simulink model "LabFabSim2022a__10_6_2023"  (R2022a)
settings: Solver=VariableStepAuto  StartTime=0.0  StopTime=400  RelTol=1e-3  EnableMultiTasking=on
model workspace (MAT data in the model file):
  JsonData : timetable (value not decoded)
  M : Simulink.Parameter (value not decoded)
  ROS_trigger = 0
  SL_ROS_VariableLengthArrays_MaxSizes : object (value not decoded)
undefined symbols (not defined in the file): DOS, DOSinitGen, DTP, DTPGen, DTPInitGen, EmptyLocFound, InitCobot, InitCobotReturn, InitializeSLD, InitLEGO, InitVGRproc2, m, MC, MCGen, MCInitGen, MO, MOGen, MOInitGen, n, NetScan, NetScanInitGen, OrderGen, Spying, SpyingInitGen, WS, WSGen, WSInitGen
libraries: sldelib x1
(part 2 of 4)

== system LabFabSim2022a__10_6_2023/NetworkScan ==
  note: Source: SLD --> Destination: Multiple
  note: Entity Gate:
      | set to open when a positive signal value is passed into the control port. Closes when negative.
  note: Recieve signal from Chance-setting Server block for activation signal
  note: Service Time: 50 Timestep
  note: Generates a single entity that causes Network Scan attack (entity generator) to generate one entity
  note: Sets NetScan_id up to 5 and resets to 1 for next NetworkScan attack
  note: On Service Completion: Send a signal to data-logging SimFunctions
  note: Service Time: 40 Timestep
  note: Service Time: 75 Timestep
  note: Service Time: 60 Timestep
  note: Service Time: 55 Timestep
  Display : Display
  Entity Gate : EntityGate  InputPortMessageModes=m,m  OutputPortMessageModes=m
  Entity Generator : EntityGenerator  InputPortMessageModes=m  OutputPortMessageModes=m  GenerationMethod=Event-based  IntergenerationTimeAction=|  GenerateAction=|  AttributeName=NetScan_id  EntityType=Structured  EntityTypeName=NetScanAttack
      IntergenerationTimeAction=|
      | chanceDOS = rand(1,1);
      | if chanceDOS < 0.3
      |     dt = 1
      GenerateAction=|
      | persistent next_id_NetScan
      | 
      | if isempty(next_id_NetScan)
      |     next_id_NetScan = 1;
      |     %set seed for random number generation
      |     rng(12345);
      | end
      | 
      | entity.NetScan_id = next_id_NetScan
      | next_id_NetScan = next_id_NetScan + 1
      | 
      | if entity.NetScan_id == 2
      |     next_id_NetScan = 1
      settings: InputPortMap=u0
  Entity Server : EntityServer  InputPortMessageModes=m  OutputPortMessageModes=m  Capacity=1  ServiceTimeValue=50  ServiceCompleteAction=|
      | sourceID(4); %sld
      | sourceAddress(7); %/sld_node
      | sourceType(1); %motion sensor
      | sourceLocation(1); %Fischertechnik
      | destinationServiceAddress(3); %/status_update (main)
      | destinationServiceType(4); %Order
      | destinationServiceLocation(1); %Fischertechnik
      | accessedNodeAddress(3); 
      | accessedNodeType(2); %Boolean
      | operation(1); %read/write
      | value(44); %none
  Entity Server1 : EntityServer  InputPortMessageModes=m  OutputPortMessageModes=m  Capacity=1  ServiceTimeValue=40  ServiceCompleteAction=|
      | sourceID(4); %sld
      | sourceAddress(7); %/sld_node
      | sourceType(1); %motion sensor
      | sourceLocation(1); %Fischertechnik
      | destinationServiceAddress(2); %/vgr_node
      | destinationServiceType(3); %Reference Switch
      | destinationServiceLocation(1); %Fischertechnik
      | accessedNodeAddress(3); 
      | accessedNodeType(2); %Boolean
      | operation(1); %read/write
      | value(44); %none
  Entity Server2 : EntityServer  InputPortMessageModes=m  OutputPortMessageModes=m  Capacity=1  ServiceTimeValue=75  ServiceCompleteAction=|
      | sourceID(4); %sld
      | sourceAddress(7); %/sld_node
      | sourceType(1); %motion sensor
      | sourceLocation(1); %Fischertechnik
      | destinationServiceAddress(4); %/lego_node
      | destinationServiceType(1); %Motion Sensor
      | destinationServiceLocation(2); %Expansion
      | accessedNodeAddress(4); 
      | accessedNodeType(1); %String
      | operation(1); %read/write
      | value(44); %none
  Entity Server3 : EntityServer  InputPortMessageModes=m  OutputPortMessageModes=m  Capacity=1  ServiceTimeValue=60  ServiceCompleteAction=|
      | sourceID(4); %sld
      | sourceAddress(7); %/sld_node
      | sourceType(1); %motion sensor
      | sourceLocation(1); %Fischertechnik
      | destinationServiceAddress(5); %/listener (cobot)
      | destinationServiceType(5); %next task
      | destinationServiceLocation(2); %Expansion
      | accessedNodeAddress(5); 
      | accessedNodeType(2); %String
      | operation(1); %read/write
      | value(44); %none
  Entity Server4 : EntityServer  InputPortMessageModes=m  OutputPortMessageModes=m  Capacity=1  ServiceTimeValue=55  ServiceCompleteAction=|
      | sourceID(4); %sld
      | sourceAddress(7); %/sld_node
      | sourceType(1); %motion sensor
      | sourceLocation(1); %Fischertechnik
      | destinationServiceAddress(1); %/hbw_node
      | destinationServiceType(4); %order
      | destinationServiceLocation(1); %Fischertechnik
      | accessedNodeAddress(7); 
      | accessedNodeType(2); %String
      | operation(1); %read/write
      | value(44); %none
  Entity Store : EntityStore  InputPortMessageModes=m  OutputPortMessageModes=m  Capacity=3
      settings: OutputPortMap=o4
  Entity Terminator1 : EntityTerminator  InputPortMessageModes=m  NumberEntitiesArrived=on
      settings: OutputPortMap=o0
  InitNetScan : Subsystem
  NetScan : Subsystem  TreatAsAtomicUnit=on
  "Number of Entities Generated from main " : Display
  Simulink Function1 : Subsystem  TreatAsAtomicUnit=on
  Subsystem1 : Subsystem
  wires:
  Simulink Function1/1(Out1) -> Entity Generator/1
  Entity Terminator1/1 -> Display/1
  Entity Generator/1 -> Entity Store/1
  Entity Store/1 -> Entity Gate/2
  Entity Server/1 -> Entity Server1/1
  NetScan/1(Out1) -> Entity Gate/1
  Subsystem1/1(Out1) -> Simulink Function1/1(In1)
  InitNetScan/1(Out1) -> "Number of Entities Generated from main "/1
  Entity Server1/1 -> Entity Server2/1
  Entity Server2/1 -> Entity Server3/1
  Entity Server3/1 -> Entity Server4/1
  Entity Server4/1 -> Entity Terminator1/1
  Entity Gate/1 -> Entity Server/1

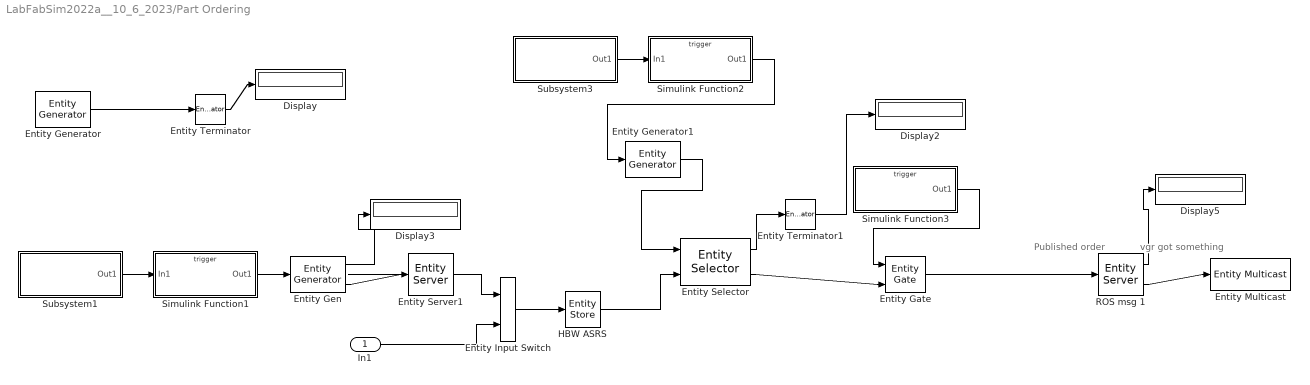
== system LabFabSim2022a__10_6_2023/Part Ordering ==
  note: vgr got something
  note: Published order
  In1 : Inport
  Display{,2..3,5} (4 alike) : Display
  Entity Input Switch : EntityInputSwitch  InputPortMessageModes=m,m  OutputPortMessageModes=m
  Entity Gate : EntityGate  InputPortMessageModes=m,m  OutputPortMessageModes=m  OperatingMode=Release gate  OpenGateAtSimulationStart=on
  "Entity Gen " : EntityGenerator  InputPortMessageModes=m  OutputPortMessageModes=n,m  GenerationMethod=Event-based  GenerateAction=|  AttributeName=PartID|ColorID|ServiceProcess|CurrentStep|CurrentRoute|HBW_ServiceTime|LEGO_ServiceTime|SLD_ServiceTime|HBW_Loc|Rand_seed  AttributeInitialValue=1|1|zeros(1,11)|0|1|zeros(1)|zeros(1)|zeros(1)|zeros(1)|1  NumberEntitiesDeparted=on  EntityType=Structured  EntityTypeName=PartOrder
      | persistent next_id
      | if isempty(next_id)
      |     next_id = 1;
      |     %set seed for random number generation
      |     rng(12345);
      | end
      | 
      | %Assign ID attribute 
      | if next_id <= 9
      |     entity.PartID = next_id;
      |     next_id = next_id + 1
      | end
      | 
      | %Current Step Attribute Setup
      | persistent SEQId;
      | persistent idx2;
      | if isempty(SEQId)
      |     SEQId = 1:15;
      |     idx2 = 1;
      | end
      | if idx2 > numel(SEQId)
      |     idx2 = 1;
      |     entity.PartID = SEQId(idx2);
      | else
      |     entity.PartID = SEQId(idx2);
      | end
      | idx2 = idx2 + 1;
      | entity.CurrentStep=1;
      | 
      | %Randomly Set Order Color 
      | entity.HBW_Loc = randi(3)
      | %To specifically select a part color, uncomment the line below and comment out the line above.
      | %entity.HBW_Loc = 3
      | switch(entity.HBW_Loc)
      |     case 1 
      |         entity.ColorID = 1;
      |         %entity.Color = "red";
      |         %red part ordered
      |     case 2
      |         entity.ColorID = 2;
      |         %entity.Color = "blue";
      |         %blue part ordered 
      |     case 3 
      |         entity.ColorID = 3;
      |         %entity.Color = "white";
      |         %white part ordered 
      | end
      | 
      | %Entity attribute based on color ID
      | if entity.ColorID == 1
      |     entity.ServiceProcess = [2 3 4 5 6 7 8 9 10 11 1];
      |     entity.HBW_ServiceTime = [5];
      |     entity.LEGO_ServiceTime = [4];
      |     entity.SLD_ServiceTime = [5];
      |     
      | else if entity.ColorID == 2
      |     entity.ServiceProcess = [2 3 4 5 6 7 8 9 10 11 1];
      |     entity.HBW_ServiceTime = [6];
      |     entity.LEGO_ServiceTime = [4];
      |     entity.SLD_ServiceTime = [4];
      |     
      | else if entity.ColorID == 3
      |     entity.ServiceProcess = [2 3 4 5 6 7 8 9 10 11 1];
      |     entity.HBW_ServiceTime = [5];
      |     entity.LEGO_ServiceTime = [6];
      |     entity.SLD_ServiceTime = [6];
      | end
      | end
      | 
      | entity.Rand_seed = 123457;
      settings: InputPortMap=u0  OutputPortMap=o0,o3
  Entity Generator : EntityGenerator  OutputPortMessageModes=m  Period=inf  AttributeName=data  EntityType=Structured  EntityTypeName=InitOrders
  Entity Generator1 : EntityGenerator  InputPortMessageModes=m  OutputPortMessageModes=m  GenerationMethod=Event-based  GenerateAction=entity.PartID = randi(9);  AttributeName=PartID  AttributeInitialValue=zeros(1)  EntityType=Structured  EntityTypeName=Order
      settings: InputPortMap=u0
  Entity Multicast : EntityMulticast  Tag=Order  InputPortMessageModes=m  MulticastTag=Order
  Entity Selector : sldelib/Entity Selector  mNumberOfStreams=1  mKeyEntityAttributeName={'PartID'}  mEntityAttributeName={'PartID'}  mMatchingNumberSource=Dialog  mNumberOfMatches=1  mNumberOfMatchesAttribute=Name  mNumEntitiesDepOpt=off  mNumEntitiesInBlockOpt=off  mNumEntitiesExtractedOpt=off
      settings: SourceProductBaseCode=SE
  Entity Server1 : EntityServer  InputPortMessageModes=m  OutputPortMessageModes=m  Capacity=1  ServiceTimeValue=0
  Entity Terminator : EntityTerminator  InputPortMessageModes=m  EntryAction=|  NumberEntitiesArrived=on
      | EntityGen();
      | EntityGen();
      | EntityGen();
      | EntityGen();
      | EntityGen();
      | EntityGen();
      | EntityGen();
      | EntityGen();
      | EntityGen();
      | 
      | %Initially set attack Routers to closed state
      | DOS_Router(2);
      | NetScan_Router(2);
      | Spying_Router(2);
      | DTP_Router(2);
      | MO_Router(2);
      | WS_Router(2);
      | MC_Router(2);
      settings: OutputPortMap=o0
  Entity Terminator1 : EntityTerminator  InputPortMessageModes=m  NumberEntitiesArrived=on
      settings: OutputPortMap=o0
  HBW ASRS : EntityStore  InputPortMessageModes=m  OutputPortMessageModes=m  Capacity=9  EntryAction=OrderGen();
      settings: OutputPortMap=o4
  ROS msg 1 : EntityServer  InputPortMessageModes=m  OutputPortMessageModes=n,m  Capacity=1  ServiceTimeSource=MATLAB action  ServiceTimeValue=0.07  ServiceTimeAction=|  EntryAction=|  ExitAction=|  NumberEntitiesDeparted=on
      ServiceTimeAction=|
      | dt=0
      | persistent rngInit;
      | if isempty(rngInit)
      |     seed = entity.Rand_seed;
      |     rng(seed);
      |     rngInit = true;
      | end
      | 
      | if entity.ColorID == 1 %red
      |     % Pattern: Uniform distribution
      |     % m: Minimum, M: Maximum
      |     m = 0.0253; M = 0.09114;
      |     dt = m + (M - m) * rand;
      | elseif entity.ColorID == 2 %blue
      |     m = 0.05309; M = 0.1517;
      |     dt = m + (M - m) * rand;
      | elseif entity.ColorID == 3 %white
      |     m = 0.06431; M = 0.24846;
      |     dt = m + (M - m) * rand;
      | end
      EntryAction=|
      | sourceID(3); %main
      | sourceAddress(6); %/order
      | sourceType(4); %order
      | sourceLocation(3); %SCADA system
      | destinationServiceAddress(1); %/hbw_node
      | destinationServiceType(4); %order
      | destinationServiceLocation(1); %Fischertechnik
      | accessedNodeAddress(7); 
      | accessedNodeType(1); %String
      | operation(3); %notify-callback
      | value(41); %Published order
      ExitAction=|
      | sourceID(3); %main
      | sourceAddress(2); %/vgr_node
      | sourceType(4); %order
      | sourceLocation(3); %SCADA system
      | destinationServiceAddress(2); %/vgr_node
      | destinationServiceType(4); %order
      | destinationServiceLocation(1); %Fischertechnik
      | accessedNodeAddress(3); 
      | accessedNodeType(1); %String
      | operation(3); %notify-callback
      | value(28); %Published order
      settings: OutputPortMap=o0,o9
  Simulink Function1 : Subsystem  TreatAsAtomicUnit=on
  Simulink Function2 : Subsystem  TreatAsAtomicUnit=on
  Simulink Function3 : Subsystem  TreatAsAtomicUnit=on
  Subsystem1 : Subsystem
  Subsystem3 : Subsystem
  wires:
  Entity Terminator/1 -> Display/1
  Subsystem1/1(Out1) -> Simulink Function1/1(In1)
  Simulink Function1/1(Out1) -> "Entity Gen "/1
  HBW ASRS/1 -> Entity Selector/2
  Simulink Function3/1(Out1) -> Entity Gate/1
  ROS msg 1/2 -> Entity Multicast/1
  ROS msg 1/1 -> Display5/1
  "Entity Gen "/1 -> Display3/1
  "Entity Gen "/2 -> Entity Server1/1
  In1/1 -> Entity Input Switch/2
  Entity Selector/1 -> Entity Terminator1/1
  Entity Generator1/1 -> Entity Selector/1
  Subsystem3/1(Out1) -> Simulink Function2/1(In1)
  Simulink Function2/1(Out1) -> Entity Generator1/1
  Entity Terminator1/1 -> Display2/1
  Entity Generator/1 -> Entity Terminator/1
  Entity Input Switch/1 -> HBW ASRS/1
  Entity Server1/1 -> Entity Input Switch/1
  Entity Selector/2 -> Entity Gate/2
  Entity Gate/1 -> ROS msg 1/1

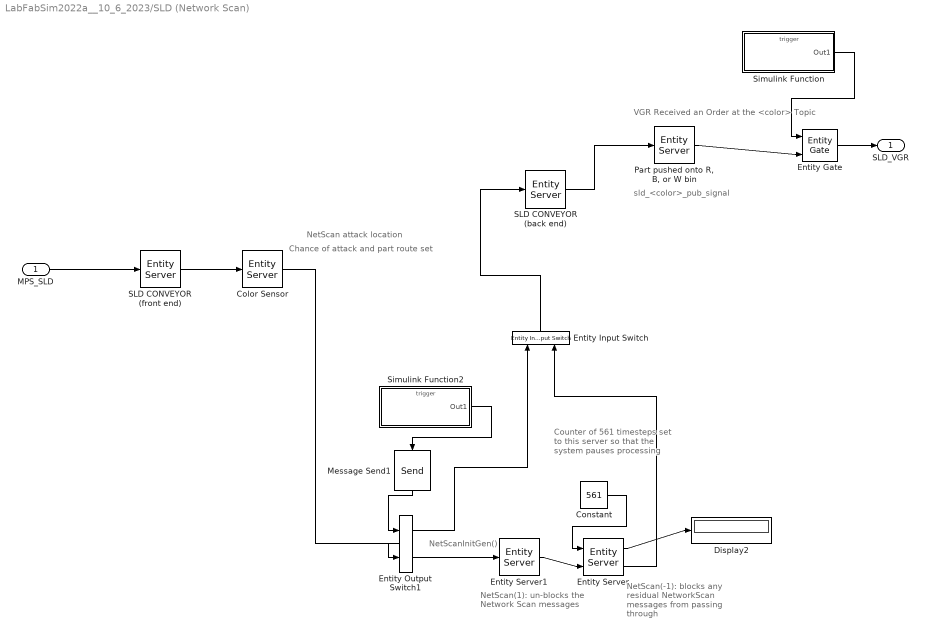
== system LabFabSim2022a__10_6_2023/SLD (Network Scan) ==
  note: VGR Received an Order at the <color> Topic
  note: sld_<color>_pub_signal
  note: NetScanInitGen()
  note: NetScan(1):
      | un-blocks the Network Scan messages
  note: NetScan(-1):
      | blocks any residual NetworkScan messages from passing through
  note: Counter of 561 timesteps set to this server so that the system pauses processing
  note: Chance of attack and part route set
  note: NetScan attack location
  MPS_SLD : Inport
  Color Sensor : EntityServer  InputPortMessageModes=m  OutputPortMessageModes=m  Capacity=1  ServiceTimeValue=0  ExitAction=|
      | chanceNetScan = rand(1,1)
      | if chanceNetScan < 0.0
      |     %Attack Happening!
      |     NetScan_Router(1);
      | 
      | else
      |     %Normal Behavior
      |     NetScan(-1);
      |     NetScan_Router(2);
      | end
  Constant : Constant  Value=561
  Display2 : Display
  Entity Input Switch : EntityInputSwitch  InputPortMessageModes=m,m  OutputPortMessageModes=m
  Entity Output Switch1 : EntityOutputSwitch  InputPortMessageModes=m,m  OutputPortMessageModes=m,m  SwitchingCriterion=From control port  SwitchAttributeName=Attribute1
      settings: InputPortMap=u0,u1
  Entity Gate : EntityGate  InputPortMessageModes=m,m  OutputPortMessageModes=m  OperatingMode=Release gate
  Entity Server : EntityServer  InputPortMessageModes=n,m  OutputPortMessageModes=n,m  Capacity=1  ServiceTimeSource=Signal port  ExitAction=NetScan(-1);  NumberEntitiesDeparted=on
      settings: InputPortMap=u0,u2  OutputPortMap=o0,o9
  Entity Server1 : EntityServer  InputPortMessageModes=m  OutputPortMessageModes=m  Capacity=1  EntryAction=NetScanInitGen();  ServiceCompleteAction=NetScan(1);
  Message Send1 : Send  OutputPortMessageModes=m
  "Part pushed onto R, B, or W bin" : EntityServer  InputPortMessageModes=m  OutputPortMessageModes=m  Capacity=1  ServiceTimeSource=MATLAB action  ServiceTimeAttributeName=SLD_ServiceTime  ServiceTimeAction=|  EntryAction=InitVGRproc2();  ExitAction=|
      ServiceTimeAction=|
      | dt=0
      | persistent rngInit;
      | if isempty(rngInit)
      |     seed = entity.Rand_seed;
      |     rng(seed);
      |     rngInit = true;
      | end
      | 
      | if entity.ColorID == 1 %red
      |     % Pattern: Uniform distribution
      |     % m: Minimum, M: Maximum
      |     m = 5.806; M = 12.40431;
      |     dt = m + (M - m) * rand;
      | elseif entity.ColorID == 2 %blue
      |     m = 13.70771; M = 15.54878;
      |     dt = m + (M - m) * rand;
      | elseif entity.ColorID == 3 %white
      |     m = 1.09164; M = 5.1134;
      |     dt = m + (M - m) * rand;
      | end
      ExitAction=|
      | sourceID(4); %sld
      | sourceAddress(7); %/vgr_node
      | sourceType(1); %motion sensor
      | sourceLocation(1); %Fischertechnik
      | destinationServiceAddress(2); %/vgr_node
      | destinationServiceType(5); %next task
      | destinationServiceLocation(1); %Fischertechnik
      | accessedNodeAddress(3); 
      | accessedNodeType(2); %String
      | operation(3); %notify-callback
      | 
      | if entity.ColorID == 1
      |     value(19); %VGR Received an Order at the RED Topic
      | else if entity.ColorID == 2
      |     value(18); %VGR Received an Order at the BLUE Topic
      | else    
      |     value(20); %VGR Received an Order at the WHITE Topic
      | end
  SLD CONVEYOR (back end) : EntityServer  InputPortMessageModes=m  OutputPortMessageModes=m  Capacity=1  ServiceTimeSource=Attribute  ServiceTimeAttributeName=SLD_ServiceTime
  SLD CONVEYOR (front end) : EntityServer  InputPortMessageModes=m  OutputPortMessageModes=m  Capacity=1  ServiceTimeValue=5
  Simulink Function : Subsystem  TreatAsAtomicUnit=on
  Simulink Function2 : Subsystem  TreatAsAtomicUnit=on
  SLD_VGR : Outport
  wires:
  MPS_SLD/1 -> SLD CONVEYOR (front end)/1
  SLD CONVEYOR (front end)/1 -> Color Sensor/1
  SLD CONVEYOR (back end)/1 -> "Part pushed onto R, B, or W bin"/1
  "Part pushed onto R, B, or W bin"/1 -> Entity Gate/2
  Entity Gate/1 -> SLD_VGR/1
  Simulink Function/1(Out1) -> Entity Gate/1
  Entity Server/1 -> Display2/1
  Entity Server1/1 -> Entity Server/2
  Entity Server/2 -> Entity Input Switch/2
  Color Sensor/1 -> Entity Output Switch1/2
  Entity Input Switch/1 -> SLD CONVEYOR (back end)/1
  Constant/1 -> Entity Server/1
  Message Send1/1 -> Entity Output Switch1/1
  Entity Output Switch1/2 -> Entity Server1/1
  Entity Output Switch1/1 -> Entity Input Switch/1
  Simulink Function2/1(Out1) -> Message Send1/1

== system LabFabSim2022a__10_6_2023/Spying ==
  note: Source: hbw --> Destination: (2,5)
  note: Entity Gate:
      | set to open when a positive signal value is passed into the control port. Closes when negative.
  note: Recieve signal from Chance-setting Server block for activation signal
  note: Service Time: 50 Timestep
  note: Generates a single entity that causes Spying attack (entity generator) to generate one entity
  note: Sets Spying_id up to 5 and resets to 1 for next Spying attack
  note: On Service Completion: Send a signal to data-logging SimFunctions
  note: Service Time: 110 Timestep
  note: Service Time: 75 Timestep
  note: Service Time: 95 Timestep
  note: Service Time: 150 Timestep
  Display : Display
  Entity Gate : EntityGate  InputPortMessageModes=m,m  OutputPortMessageModes=m
  Entity Generator : EntityGenerator  InputPortMessageModes=m  OutputPortMessageModes=m  GenerationMethod=Event-based  IntergenerationTimeAction=|  GenerateAction=|  AttributeName=Spying_id  EntityType=Structured  EntityTypeName=SpyingAttack
      IntergenerationTimeAction=|
      | chanceDOS = rand(1,1);
      | if chanceDOS < 0.3
      |     dt = 1
      GenerateAction=|
      | persistent next_id_Spying
      | 
      | if isempty(next_id_Spying)
      |     next_id_Spying = 1;
      |     %set seed for random number generation
      |     rng(12345);
      | end
      | 
      | entity.Spying_id = next_id_Spying
      | next_id_Spying = next_id_Spying + 1
      | 
      | if entity.Spying_id == 5
      |     next_id_Spying = 1
      settings: InputPortMap=u0
  Entity Server : EntityServer  InputPortMessageModes=m  OutputPortMessageModes=m  Capacity=1  ServiceTimeValue=50  ServiceCompleteAction=|
      | sourceID(1); %hbw
      | sourceAddress(1); %/hbw_node
      | sourceType(5); %next_task
      | sourceLocation(1); %Fischertechnik
      | destinationServiceAddress(2); %/vgr_node
      | destinationServiceType(1); %Motion Sensor
      | destinationServiceLocation(1); %Fischertechnik
      | accessedNodeAddress(3); 
      | accessedNodeType(2); %Boolean
      | operation(1); %read/write
      | value(45); %Spy
  Entity Server1 : EntityServer  InputPortMessageModes=m  OutputPortMessageModes=m  Capacity=1  ServiceTimeValue=110  ServiceCompleteAction=|
      | sourceID(1); %hbw
      | sourceAddress(1); %/hbw_node
      | sourceType(5); %next_task
      | sourceLocation(1); %Fischertechnik
      | destinationServiceAddress(5); %/lego_node
      | destinationServiceType(1); %Motion Sensor
      | destinationServiceLocation(2); %Expansion
      | accessedNodeAddress(5); 
      | accessedNodeType(2); %Boolean
      | operation(1); %read/write
      | value(45); %Spy
  Entity Server2 : EntityServer  InputPortMessageModes=m  OutputPortMessageModes=m  Capacity=1  ServiceTimeValue=75  ServiceCompleteAction=|
      | sourceID(1); %hbw
      | sourceAddress(1); %/hbw_node
      | sourceType(5); %next_task
      | sourceLocation(1); %Fischertechnik
      | destinationServiceAddress(2); %/vgr_node
      | destinationServiceType(1); %Motion Sensor
      | destinationServiceLocation(1); %Fischertechnik
      | accessedNodeAddress(3); 
      | accessedNodeType(2); %Boolean
      | operation(1); %read/write
      | value(45); %Spy
  Entity Server3 : EntityServer  InputPortMessageModes=m  OutputPortMessageModes=m  Capacity=1  ServiceTimeValue=95  ServiceCompleteAction=|
      | sourceID(1); %hbw
      | sourceAddress(1); %/hbw_node
      | sourceType(5); %next_task
      | sourceLocation(1); %Fischertechnik
      | destinationServiceAddress(5); %/lego_node
      | destinationServiceType(1); %Motion Sensor
      | destinationServiceLocation(2); %Expansion
      | accessedNodeAddress(5);  
      | accessedNodeType(2); %Boolean
      | operation(1); %read/write
      | value(45); %Spy
  Entity Server4 : EntityServer  InputPortMessageModes=m  OutputPortMessageModes=m  Capacity=1  ServiceTimeValue=150  ServiceCompleteAction=|
      | sourceID(1); %hbw
      | sourceAddress(1); %/hbw_node
      | sourceType(5); %next_task
      | sourceLocation(1); %Fischertechnik
      | destinationServiceAddress(5); %/lego_node
      | destinationServiceType(1); %Motion Sensor
      | destinationServiceLocation(2); %Expansion
      | accessedNodeAddress(5);  
      | accessedNodeType(2); %Boolean
      | operation(1); %read/write
      | value(45); %Spy
  Entity Store : EntityStore  InputPortMessageModes=m  OutputPortMessageModes=m  Capacity=6
      settings: OutputPortMap=o4
  Entity Terminator1 : EntityTerminator  InputPortMessageModes=m  NumberEntitiesArrived=on
      settings: OutputPortMap=o0
  InitSpying : Subsystem
  "Number of Entities Generated from main " : Display
  Simulink Function1 : Subsystem  TreatAsAtomicUnit=on
  Spying : Subsystem  TreatAsAtomicUnit=on
  Subsystem1 : Subsystem
  wires:
  Simulink Function1/1(Out1) -> Entity Generator/1
  Entity Terminator1/1 -> Display/1
  Entity Generator/1 -> Entity Store/1
  Entity Store/1 -> Entity Gate/2
  Entity Server/1 -> Entity Server1/1
  Spying/1(Out1) -> Entity Gate/1
  Subsystem1/1(Out1) -> Simulink Function1/1(In1)
  InitSpying/1(Out1) -> "Number of Entities Generated from main "/1
  Entity Server1/1 -> Entity Server2/1
  Entity Server2/1 -> Entity Server3/1
  Entity Server3/1 -> Entity Server4/1
  Entity Server4/1 -> Entity Terminator1/1
  Entity Gate/1 -> Entity Server/1

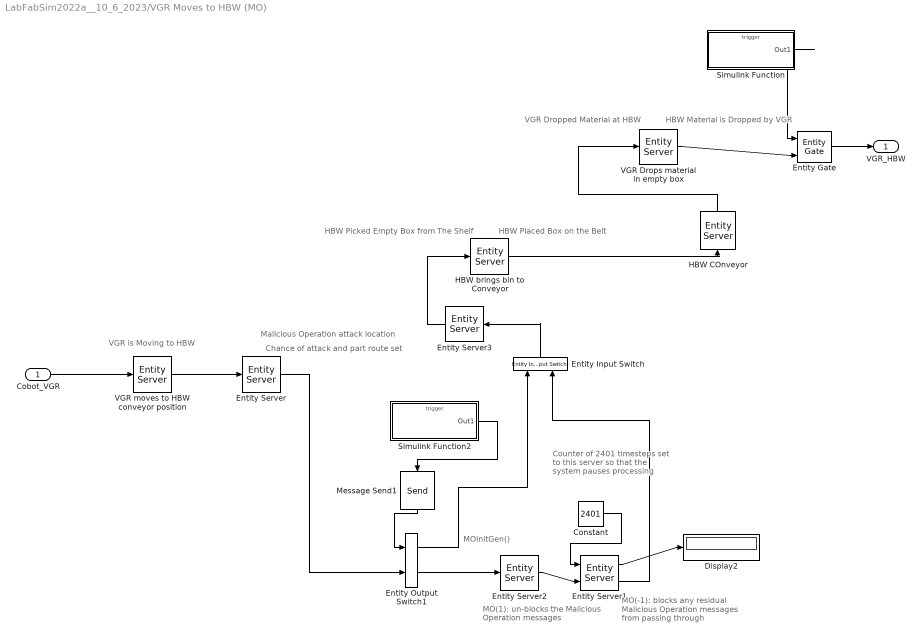
== system LabFabSim2022a__10_6_2023/VGR Moves to HBW (MO) ==
  note: HBW Material is Dropped by VGR
  note: VGR Dropped Material at HBW
  note: HBW Placed Box on the Belt
  note: HBW Picked Empty Box from The Shelf
  note: VGR is Moving to HBW
  note: MOInitGen()
  note: MO(-1):
      | blocks any residual Malicious Operation messages from passing through
  note: MO(1):
      | un-blocks the Malicious Operation messages
  note: Counter of 2401 timesteps set to this server so that the system pauses processing
  note: Malicious Operation attack location
  note: Chance of attack and part route set
  Cobot_VGR : Inport
  Constant : Constant  Value=2401
  Display2 : Display
  Entity Input Switch : EntityInputSwitch  InputPortMessageModes=m,m  OutputPortMessageModes=m
  Entity Output Switch1 : EntityOutputSwitch  InputPortMessageModes=m,m  OutputPortMessageModes=m,m  SwitchingCriterion=From control port  SwitchAttributeName=Attribute1
      settings: InputPortMap=u0,u1
  Entity Gate : EntityGate  InputPortMessageModes=m,m  OutputPortMessageModes=m  OperatingMode=Release gate
  Entity Server : EntityServer  InputPortMessageModes=m  OutputPortMessageModes=m  Capacity=1  ServiceTimeValue=0  ExitAction=|
      | chanceMO = rand(1,1)
      | if chanceMO < 0.0
      |     %Attack Happening!
      |     MO_Router(1);
      | 
      | else
      |     %Normal Behavior
      |     MO(-1);
      |     MO_Router(2);
      | end
  Entity Server1 : EntityServer  InputPortMessageModes=n,m  OutputPortMessageModes=n,m  Capacity=1  ServiceTimeSource=Signal port  ExitAction=MO(-1);  NumberEntitiesDeparted=on
      settings: InputPortMap=u0,u2  OutputPortMap=o0,o9
  Entity Server2 : EntityServer  InputPortMessageModes=m  OutputPortMessageModes=m  Capacity=1  EntryAction=MOInitGen();  ServiceCompleteAction=MO(1);
  Entity Server3 : EntityServer  InputPortMessageModes=m  OutputPortMessageModes=m  Capacity=1  ServiceTimeSource=MATLAB action  ServiceTimeAction=|
      | dt=0
      | persistent rngInit;
      | if isempty(rngInit)
      |     seed = entity.Rand_seed;
      |     rng(seed);
      |     rngInit = true;
      | end
      | 
      | if entity.ColorID == 1 %red
      |     % Pattern: Uniform distribution
      |     % m: Minimum, M: Maximum
      |     m = 9.7679; M = 9.7679;
      |     dt = m + (M - m) * rand;
      | elseif entity.ColorID == 2 %blue
      |     m = 6.5315; M = 7.32;
      |     dt = m + (M - m) * rand;
      | elseif entity.ColorID == 3 %white
      |     m = 13.1578; M = 13.8905;
      |     dt = m + (M - m) * rand;
      | end
  HBW COnveyor : EntityServer  InputPortMessageModes=m  OutputPortMessageModes=m  Capacity=1  ServiceTimeSource=MATLAB action  ServiceTimeAction=|
      | dt=0
      | persistent rngInit;
      | if isempty(rngInit)
      |     seed = entity.Rand_seed;
      |     rng(seed);
      |     rngInit = true;
      | end
      | 
      | if entity.ColorID == 1 %red
      |     % Pattern: Uniform distribution
      |     % m: Minimum, M: Maximum
      |     m = 0.0599; M = 0.7454;
      |     dt = m + (M - m) * rand;
      | elseif entity.ColorID == 2 %blue
      |     m = 0.6055; M = 0.6167;
      |     dt = m + (M - m) * rand;
      | elseif entity.ColorID == 3 %white
      |     m = 0.6407; M = 0.6611;
      |     dt = m + (M - m) * rand;
      | end
  HBW brings bin to Conveyor : EntityServer  InputPortMessageModes=m  OutputPortMessageModes=m  Capacity=1  ServiceTimeSource=MATLAB action  ServiceTimeValue=3  ServiceTimeAttributeName=HBW_ServiceTime  ServiceTimeAction=|  EntryAction=|  ExitAction=|
      ServiceTimeAction=|
      | dt=0
      | persistent rngInit;
      | if isempty(rngInit)
      |     seed = entity.Rand_seed;
      |     rng(seed);
      |     rngInit = true;
      | end
      | 
      | if entity.ColorID == 1 %red
      |     % Pattern: Uniform distribution
      |     % m: Minimum, M: Maximum
      |     m = 20.0831; M = 20.9407;
      |     dt = m + (M - m) * rand;
      | elseif entity.ColorID == 2 %blue
      |     m = 17.0487; M = 17.2651;
      |     dt = m + (M - m) * rand;
      | elseif entity.ColorID == 3 %white
      |     m = 23.2158; M = 24.0842;
      |     dt = m + (M - m) * rand;
      | end
      EntryAction=|
      | sourceID(1); %hbw
      | sourceAddress(1); %/hbw_node
      | sourceType(3); %reference switch
      | sourceLocation(1); %Fischertechnik
      | destinationServiceAddress(1); %/hbw_node
      | destinationServiceType(5); %next task
      | destinationServiceLocation(1); %Fischertechnik
      | accessedNodeAddress(1); 
      | accessedNodeType(1); %String
      | operation(3); %notify-callback
      | value(4); %HBW Picked Empty Box from The Shelf
      ExitAction=|
      | sourceID(1); %hbw
      | sourceAddress(1); %/hbw_node
      | sourceType(1); %Motion Sensor
      | sourceLocation(1); %Fischertechnik
      | destinationServiceAddress(1); %/hbw_node
      | destinationServiceType(5); %next task
      | destinationServiceLocation(1); %Fischertechnik
      | accessedNodeAddress(1); 
      | accessedNodeType(1); %String
      | operation(3); %notify-callback
      | value(6); %HBW Placed Box on the Belt
  Message Send1 : Send  OutputPortMessageModes=m
  Simulink Function : Subsystem  TreatAsAtomicUnit=on
  Simulink Function2 : Subsystem  TreatAsAtomicUnit=on
  VGR Drops material in empty box : EntityServer  InputPortMessageModes=m  OutputPortMessageModes=m  Capacity=1  ServiceTimeSource=MATLAB action  ServiceTimeValue=6  ServiceTimeAttributeName=HBW_ServiceTime  ServiceTimeAction=|  EntryAction=|  ExitAction=|
      ServiceTimeAction=|
      | dt=0
      | persistent rngInit;
      | if isempty(rngInit)
      |     seed = entity.Rand_seed;
      |     rng(seed);
      |     rngInit = true;
      | end
      | 
      | if entity.ColorID == 1 %red
      |     % Pattern: Uniform distribution
      |     % m: Minimum, M: Maximum
      |     m = 6.1187; M = 6.3253;
      |     dt = m + (M - m) * rand;
      | elseif entity.ColorID == 2 %blue
      |     m = 6.3414; M = 6.4349;
      |     dt = m + (M - m) * rand;
      | elseif entity.ColorID == 3 %white
      |     m = 6.3623; M = 6.4411;
      |     dt = m + (M - m) * rand;
      | end
      EntryAction=|
      | BinSupplied();
      | 
      | sourceID(1); %hbw
      | sourceAddress(1); %/hbw_node
      | sourceType(1); %Motion Sensor 
      | sourceLocation(1); %Fischertechnik
      | destinationServiceAddress(2); %/vgr_node
      | destinationServiceType(5); %next task
      | destinationServiceLocation(1); %Fischertechnik
      | accessedNodeAddress(3); 
      | accessedNodeType(2); %Boolean
      | operation(3); %notify-callback
      | value(21); %VGR Dropped Material at HBW
      ExitAction=|
      | sourceID(1); %hbw
      | sourceAddress(1); %/hbw_node
      | sourceType(5); %next task
      | sourceLocation(1); %Fischertechnik
      | destinationServiceAddress(1); %/hbw_node
      | destinationServiceType(5); %next task
      | destinationServiceLocation(1); %Fischertechnik
      | accessedNodeAddress(1); 
      | accessedNodeType(1); %String
      | operation(3); %notify-callback
      | value(8); %HBW Material is Dropped by VGR
  VGR moves to HBW conveyor position : EntityServer  InputPortMessageModes=m  OutputPortMessageModes=m  Capacity=1  ServiceTimeSource=MATLAB action  ServiceTimeValue=3  ServiceTimeAction=|  ServiceCompleteAction=|
      ServiceTimeAction=|
      | dt=0
      | persistent rngInit;
      | if isempty(rngInit)
      |     seed = entity.Rand_seed;
      |     rng(seed);
      |     rngInit = true;
      | end
      | 
      | if entity.ColorID == 1 %red
      |     % Pattern: Uniform distribution
      |     % m: Minimum, M: Maximum
      |     m = 9.1993; M = 9.5444;
      |     dt = m + (M - m) * rand;
      | elseif entity.ColorID == 2 %blue
      |     m = 8.5836; M = 9.294;
      |     dt = m + (M - m) * rand;
      | elseif entity.ColorID == 3 %white
      |     m = 9.1114; M = 9.2737;
      |     dt = m + (M - m) * rand;
      | end
      ServiceCompleteAction=|
      | sourceID(3); %main
      | sourceAddress(6); %/order
      | sourceType(5); %next task
      | sourceLocation(1); %Fischer
      | destinationServiceAddress(2); %/vgr_node
      | destinationServiceType(5); %next task
      | destinationServiceLocation(1); %Fischertechnik
      | accessedNodeAddress(3); 
      | accessedNodeType(1); %String
      | operation(3); %notify-callback
      | value(29); %vgr is moving to hbw
  VGR_HBW : Outport
  wires:
  VGR moves to HBW conveyor position/1 -> Entity Server/1
  Cobot_VGR/1 -> VGR moves to HBW conveyor position/1
  Entity Gate/1 -> VGR_HBW/1
  Simulink Function/1(Out1) -> Entity Gate/1
  VGR Drops material in empty box/1 -> Entity Gate/2
  HBW brings bin to Conveyor/1 -> HBW COnveyor/1
  Entity Server1/1 -> Display2/1
  Constant/1 -> Entity Server1/1
  Entity Input Switch/1 -> Entity Server3/1
  Entity Server/1 -> Entity Output Switch1/2
  Entity Output Switch1/2 -> Entity Server2/1
  Simulink Function2/1(Out1) -> Message Send1/1
  Entity Server2/1 -> Entity Server1/2
  Entity Server1/2 -> Entity Input Switch/2
  Message Send1/1 -> Entity Output Switch1/1
  Entity Output Switch1/1 -> Entity Input Switch/1
  Entity Server3/1 -> HBW brings bin to Conveyor/1
  HBW COnveyor/1 -> VGR Drops material in empty box/1

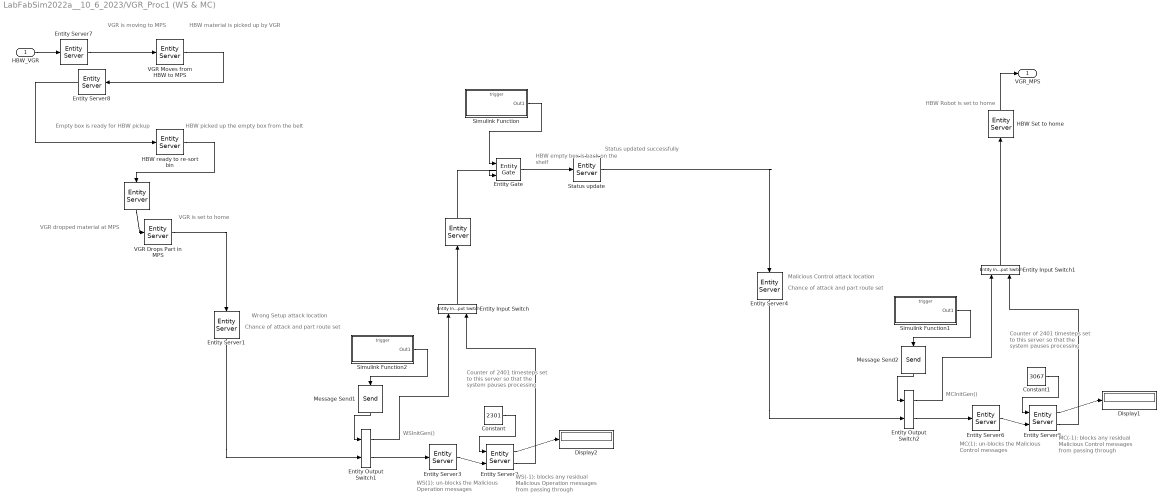
== system LabFabSim2022a__10_6_2023/VGR_Proc1 (WS & MC) ==
  note: Status updated successfully
  note: HBW empty box is back on the shelf
  note: HBW Robot is set to home
  note: VGR is set to home
  note: VGR dropped material at MPS
  note: HBW picked up the empty box from the belt
  note: Empty box is ready for HBW pickup
  note: HBW material is picked up by VGR
  note: VGR is moving to MPS
  note: WS(-1):
      | blocks any residual Malicious Operation messages from passing through
  note: Counter of 2401 timesteps set to this server so that the system pauses processing
  note: Chance of attack and part route set
  note: WSInitGen()
  note: WS(1):
      | un-blocks the Malicious Operation messages
  note: Wrong Setup attack location
  note: MC(-1):
      | blocks any residual Malicious Control messages from passing through
  note: MCInitGen()
  note: Chance of attack and part route set
  note: Malicious Control attack location
  note: Counter of 2401 timesteps set to this server so that the system pauses processing
  note: MC(1):
      | un-blocks the Malicious Control messages
  HBW_VGR : Inport
  " " : EntityServer  InputPortMessageModes=m  OutputPortMessageModes=m  Capacity=1  ServiceTimeSource=MATLAB action  ServiceTimeValue=10.5  ServiceTimeAction=|
      | dt=0
      | persistent rngInit;
      | if isempty(rngInit)
      |     seed = entity.Rand_seed;
      |     rng(seed);
      |     rngInit = true;
      | end
      | 
      | if entity.ColorID == 1 %red
      |     % Pattern: Uniform distribution
      |     % m: Minimum, M: Maximum
      |     m = 9.76528; M = 9.92263;
      |     dt = m + (M - m) * rand;
      | elseif entity.ColorID == 2 %blue
      |     m = 9.79401; M = 9.93601;
      |     dt = m + (M - m) * rand;
      | elseif entity.ColorID == 3 %white
      |     m = 9.8831; M = 9.99734;
      |     dt = m + (M - m) * rand;
      | end
  "   " : EntityServer  InputPortMessageModes=m  OutputPortMessageModes=m  Capacity=1  ServiceTimeSource=MATLAB action  ServiceTimeValue=10.5  ServiceTimeAction=|
      | dt=0
      | persistent rngInit;
      | if isempty(rngInit)
      |     seed = entity.Rand_seed;
      |     rng(seed);
      |     rngInit = true;
      | end
      | 
      | if entity.ColorID == 1 %red
      |     % Pattern: Uniform distribution
      |     % m: Minimum, M: Maximum
      |     m = 9.63801; M = 11.36774;
      |     dt = m + (M - m) * rand;
      | elseif entity.ColorID == 2 %blue
      |     m = 8.05698; M = 8.4006;
      |     dt = m + (M - m) * rand;
      | elseif entity.ColorID == 3 %white
      |     m = 14.757; M = 15.37227;
      |     dt = m + (M - m) * rand;
      | end
  Constant : Constant  Value=2301
  Constant1 : Constant  Value=3067
  Display1 : Display
  Display2 : Display
  Entity Input Switch : EntityInputSwitch  InputPortMessageModes=m,m  OutputPortMessageModes=m
  Entity Input Switch1 : EntityInputSwitch  InputPortMessageModes=m,m  OutputPortMessageModes=m
  Entity Output Switch1 : EntityOutputSwitch  InputPortMessageModes=m,m  OutputPortMessageModes=m,m  SwitchingCriterion=From control port  SwitchAttributeName=Attribute1
      settings: InputPortMap=u0,u1
  Entity Output Switch2 : EntityOutputSwitch  InputPortMessageModes=m,m  OutputPortMessageModes=m,m  SwitchingCriterion=From control port  SwitchAttributeName=Attribute1
      settings: InputPortMap=u0,u1
  Entity Gate : EntityGate  InputPortMessageModes=m,m  OutputPortMessageModes=m  OperatingMode=Release gate
  Entity Server1 : EntityServer  InputPortMessageModes=m  OutputPortMessageModes=m  Capacity=1  ServiceTimeValue=0  ExitAction=|
      | chanceWS = rand(1,1)
      | if chanceWS < 0.0
      |     %Attack Happening!
      |     WS_Router(1);
      | 
      | else
      |     %Normal Behavior
      |     WS(-1);
      |     WS_Router(2);
      | end
  Entity Server2 : EntityServer  InputPortMessageModes=n,m  OutputPortMessageModes=n,m  Capacity=1  ServiceTimeSource=Signal port  ExitAction=WS(-1);  NumberEntitiesDeparted=on
      settings: InputPortMap=u0,u2  OutputPortMap=o0,o9
  Entity Server3 : EntityServer  InputPortMessageModes=m  OutputPortMessageModes=m  Capacity=1  EntryAction=WSInitGen();  ServiceCompleteAction=WS(1);
  Entity Server4 : EntityServer  InputPortMessageModes=m  OutputPortMessageModes=m  Capacity=1  ServiceTimeValue=0  ExitAction=|
      | chanceMC = rand(1,1)
      | if chanceMC < 0.0
      |     %Attack Happening!
      |     MC_Router(1);
      | 
      | else
      |     %Normal Behavior
      |     MC(-1);
      |     MC_Router(2);
      | end
  Entity Server5 : EntityServer  InputPortMessageModes=n,m  OutputPortMessageModes=n,m  Capacity=1  ServiceTimeSource=Signal port  ExitAction=MC(-1);  NumberEntitiesDeparted=on
      settings: InputPortMap=u0,u2  OutputPortMap=o0,o9
  Entity Server6 : EntityServer  InputPortMessageModes=m  OutputPortMessageModes=m  Capacity=1  EntryAction=MCInitGen();  ServiceCompleteAction=MC(1);
  Entity Server7 : EntityServer  InputPortMessageModes=m  OutputPortMessageModes=m  Capacity=1  ServiceTimeSource=MATLAB action  ServiceTimeValue=10.5  ServiceTimeAction=|
      | dt=0
      | persistent rngInit;
      | if isempty(rngInit)
      |     seed = entity.Rand_seed;
      |     rng(seed);
      |     rngInit = true;
      | end
      | 
      | if entity.ColorID == 1 %red
      |     % Pattern: Uniform distribution
      |     % m: Minimum, M: Maximum
      |     m = 0.00935; M = 0.02417;
      |     dt = m + (M - m) * rand;
      | elseif entity.ColorID == 2 %blue
      |     m = 0.0089; M = 0.00966;
      |     dt = m + (M - m) * rand;
      | elseif entity.ColorID == 3 %white
      |     m = 0.00819; M = 0.01182;
      |     dt = m + (M - m) * rand;
      | end
  Entity Server8 : EntityServer  InputPortMessageModes=m  OutputPortMessageModes=m  Capacity=1  ServiceTimeSource=MATLAB action  ServiceTimeValue=10.5  ServiceTimeAction=|
      | dt=0
      | persistent rngInit;
      | if isempty(rngInit)
      |     seed = entity.Rand_seed;
      |     rng(seed);
      |     rngInit = true;
      | end
      | 
      | if entity.ColorID == 1 %red
      |     % Pattern: Uniform distribution
      |     % m: Minimum, M: Maximum
      |     m = 1.99938; M = 2.0016;
      |     dt = m + (M - m) * rand;
      | elseif entity.ColorID == 2 %blue
      |     m = 1.99838; M = 2.20301;
      |     dt = m + (M - m) * rand;
      | elseif entity.ColorID == 3 %white
      |     m = 1.96445; M = 2.01255;
      |     dt = m + (M - m) * rand;
      | end
  HBW Set to home : EntityServer  InputPortMessageModes=m  OutputPortMessageModes=m  Capacity=1  ServiceTimeSource=MATLAB action  ServiceTimeValue=14.5  ServiceTimeAction=|  ExitAction=|
      ServiceTimeAction=|
      | dt=0
      | persistent rngInit;
      | if isempty(rngInit)
      |     seed = entity.Rand_seed;
      |     rng(seed);
      |     rngInit = true;
      | end
      | 
      | if entity.ColorID == 1 %red
      |     % Pattern: Uniform distribution
      |     % m: Minimum, M: Maximum
      |     m = 8.95817; M = 9.17969;
      |     dt = m + (M - m) * rand;
      | elseif entity.ColorID == 2 %blue
      |     m = 3.05638; M = 3.55072;
      |     dt = m + (M - m) * rand;
      | elseif entity.ColorID == 3 %white
      |     m = 15.575; M = 16.95394;
      |     dt = m + (M - m) * rand;
      | end
      ExitAction=|
      | sourceID(1); %hbw
      | sourceAddress(1); %/hbw_node
      | sourceType(3); %reference switch
      | sourceLocation(1); %Fischertechnik
      | destinationServiceAddress(3); %/status_update
      | destinationServiceType(5); %next task
      | destinationServiceLocation(1); %Fischertechnik
      | accessedNodeAddress(1); 
      | accessedNodeType(1); %String
      | operation(3); %notify-callback
      | value(15); %hbw robot is set to home
  HBW ready to re-sort bin : EntityServer  InputPortMessageModes=m  OutputPortMessageModes=m  Capacity=1  ServiceTimeSource=MATLAB action  ServiceTimeValue=2  ServiceTimeAction=|  EntryAction=|  ExitAction=|
      ServiceTimeAction=|
      | dt=0
      | persistent rngInit;
      | if isempty(rngInit)
      |     seed = entity.Rand_seed;
      |     rng(seed);
      |     rngInit = true;
      | end
      | 
      | if entity.ColorID == 1 %red
      |     % Pattern: Uniform distribution
      |     % m: Minimum, M: Maximum
      |     m = 0.53151; M = 0.54027;
      |     dt = m + (M - m) * rand;
      | elseif entity.ColorID == 2 %blue
      |     m = 0.35447; M = 0.56167;
      |     dt = m + (M - m) * rand;
      | elseif entity.ColorID == 3 %white
      |     m = 0.51454; M = 0.56926;
      |     dt = m + (M - m) * rand;
      | end
      EntryAction=|
      | sourceID(1); %hbw
      | sourceAddress(1); %/hbw_node
      | sourceType(1); %Motion Sensor
      | sourceLocation(1); %Fischertechnik
      | destinationServiceAddress(1); %/hbw_node
      | destinationServiceType(5); %next task
      | destinationServiceLocation(1); %Fischertechnik
      | accessedNodeAddress(1); 
      | accessedNodeType(1); %String
      | operation(3); %notify-callback
      | value(9); %Empty box is ready for HBW pickup
      ExitAction=|
      | sourceID(1); %hbw
      | sourceAddress(1); %/hbw_node
      | sourceType(5); %next task
      | sourceLocation(1); %Fischertechnik
      | destinationServiceAddress(1); %/hbw_node
      | destinationServiceType(5); %next task
      | destinationServiceLocation(1); %Fischertechnik
      | accessedNodeAddress(1); 
      | accessedNodeType(1); %String
      | operation(3); %notify-callback
      | value(11); %hbw picked up the empty box from the beltt
  Message Send1 : Send  OutputPortMessageModes=m
  Message Send2 : Send  OutputPortMessageModes=m
  Simulink Function : Subsystem  TreatAsAtomicUnit=on
  Simulink Function1 : Subsystem  TreatAsAtomicUnit=on
  Simulink Function2 : Subsystem  TreatAsAtomicUnit=on
  Status update : EntityServer  InputPortMessageModes=m  OutputPortMessageModes=m  Capacity=1  ServiceTimeSource=MATLAB action  ServiceTimeValue=0.5  ServiceTimeAction=|  EntryAction=|  ExitAction=|
      ServiceTimeAction=|
      | dt=0
      | persistent rngInit;
      | if isempty(rngInit)
      |     seed = entity.Rand_seed;
      |     rng(seed);
      |     rngInit = true;
      | end
      | 
      | if entity.ColorID == 1 %red
      |     % Pattern: Uniform distribution
      |     % m: Minimum, M: Maximum
      |     m = 0.01118; M = 0.31391;
      |     dt = m + (M - m) * rand;
      | elseif entity.ColorID == 2 %blue
      |     m = 0.0136; M = 0.02573;
      |     dt = m + (M - m) * rand;
      | elseif entity.ColorID == 3 %white
      |     m = 0.00347; M = 0.01262;
      |     dt = m + (M - m) * rand;
      | end
      EntryAction=|
      | sourceID(1); %hbw
      | sourceAddress(1); %/hbw_node
      | sourceType(5); %next task
      | sourceLocation(1); %Fischertechnik
      | destinationServiceAddress(3); %/status_update
      | destinationServiceType(5); %next task
      | destinationServiceLocation(1); %Fischertechnik
      | accessedNodeAddress(1); 
      | accessedNodeType(1); %String
      | operation(3); %notify-callback
      | value(13); %hbw empty box is back on the shelf
      ExitAction=|
      | sourceID(1); %hbw
      | sourceAddress(1); %/hbw_node
      | sourceType(5); %next task
      | sourceLocation(1); %Fischertechnik
      | destinationServiceAddress(3); %/status_update
      | destinationServiceType(5); %next task
      | destinationServiceLocation(1); %Fischertechnik
      | accessedNodeAddress(6); 
      | accessedNodeType(1); %String
      | operation(3); %notify-callback
      | value(42); %Status Updated Successfully
  VGR Drops Part in MPS : EntityServer  InputPortMessageModes=m  OutputPortMessageModes=m  Capacity=1  ServiceTimeSource=MATLAB action  ServiceTimeValue=15.5  ServiceTimeAction=|  EntryAction=|  ExitAction=|
      ServiceTimeAction=|
      | dt=0
      | persistent rngInit;
      | if isempty(rngInit)
      |     seed = entity.Rand_seed;
      |     rng(seed);
      |     rngInit = true;
      | end
      | 
      | if entity.ColorID == 1 %red
      |     % Pattern: Uniform distribution
      |     % m: Minimum, M: Maximum
      |     m = 4.07551; M = 5.40165;
      |     dt = m + (M - m) * rand;
      | elseif entity.ColorID == 2 %blue
      |     m = 6.84048; M = 7.44307;
      |     dt = m + (M - m) * rand;
      | elseif entity.ColorID == 3 %white
      |     m = 0.01944; M = 0.66827;
      |     dt = m + (M - m) * rand;
      | end
      EntryAction=|
      | MPS_Initialize();
      | 
      | sourceID(2); %vgr
      | sourceAddress(2); %/vgr_node
      | sourceType(5); %next task
      | sourceLocation(1); %Fischertechnik
      | destinationServiceAddress(2); %/vgr_node
      | destinationServiceType(1); %motion sensor
      | destinationServiceLocation(1); %Fischertechnik
      | accessedNodeAddress(3); 
      | accessedNodeType(1); %String
      | operation(3); %notify-callback
      | value(32); %vgr dropped material at MPS
      ExitAction=|
      | sourceID(2); %vgr
      | sourceAddress(2); %/vgr_node
      | sourceType(5); %next task
      | sourceLocation(1); %Fischertechnik
      | destinationServiceAddress(2); %/vgr_node
      | destinationServiceType(3); %reference switch
      | destinationServiceLocation(1); %Fischertechnik
      | accessedNodeAddress(3); 
      | accessedNodeType(1); %String
      | operation(3); %notify-callback
      | value(16); %vgr is set to home
  VGR Moves from HBW to MPS : EntityServer  InputPortMessageModes=m  OutputPortMessageModes=m  Capacity=1  ServiceTimeSource=MATLAB action  ServiceTimeValue=1.5  ServiceTimeAction=|  EntryAction=|  ExitAction=|
      ServiceTimeAction=|
      | dt=0
      | persistent rngInit;
      | if isempty(rngInit)
      |     seed = entity.Rand_seed;
      |     rng(seed);
      |     rngInit = true;
      | end
      | 
      | if entity.ColorID == 1 %red
      |     % Pattern: Uniform distribution
      |     % m: Minimum, M: Maximum
      |     m = 1.96446; M = 2.03648;
      |     dt = m + (M - m) * rand;
      | elseif entity.ColorID == 2 %blue
      |     m = 1.91392; M = 1.96192;
      |     dt = m + (M - m) * rand;
      | elseif entity.ColorID == 3 %white
      |     m = 2.02142; M = 2.03783;
      |     dt = m + (M - m) * rand;
      | end
      EntryAction=|
      | sourceID(2); %vgr
      | sourceAddress(2); %/vgr_node
      | sourceType(3); %reference switch
      | sourceLocation(1); %Fischertechnik
      | destinationServiceAddress(2); %/vgr_node
      | destinationServiceType(5); %next task
      | destinationServiceLocation(1); %Fischertechnik
      | accessedNodeAddress(3); 
      | accessedNodeType(1); %String
      | operation(3); %notify-callback
      | value(31); %VGR is moving to MPS
      ExitAction=|
      | sourceID(1); %hbw
      | sourceAddress(1); %/hbw_node
      | sourceType(5); %next task
      | sourceLocation(1); %Fischertechnik
      | destinationServiceAddress(1); %/hbw_node
      | destinationServiceType(5); %next task
      | destinationServiceLocation(1); %Fischertechnik
      | accessedNodeAddress(1); 
      | accessedNodeType(1); %String
      | operation(3); %notify-callback
      | value(7); %hbw material is picked up by vgr
  VGR_MPS : Outport
  wires:
  Simulink Function/1(Out1) -> Entity Gate/1
  VGR Moves from HBW to MPS/1 -> Entity Server8/1
  HBW ready to re-sort bin/1 -> " "/1
  HBW_VGR/1 -> Entity Server7/1
  VGR Drops Part in MPS/1 -> Entity Server1/1
  Entity Gate/1 -> Status update/1
  HBW Set to home/1 -> VGR_MPS/1
  " "/1 -> VGR Drops Part in MPS/1
  Entity Input Switch/1 -> "   "/1
  Entity Server1/1 -> Entity Output Switch1/2
  Entity Server3/1 -> Entity Server2/2
  Simulink Function2/1(Out1) -> Message Send1/1
  Entity Output Switch1/1 -> Entity Input Switch/1
  Message Send1/1 -> Entity Output Switch1/1
  Entity Server2/2 -> Entity Input Switch/2
  Entity Output Switch1/2 -> Entity Server3/1
  Constant/1 -> Entity Server2/1
  Entity Server2/1 -> Display2/1
  Status update/1 -> Entity Server4/1
  Entity Input Switch1/1 -> HBW Set to home/1
  Entity Server5/1 -> Display1/1
  Entity Server4/1 -> Entity Output Switch2/2
  Entity Output Switch2/2 -> Entity Server6/1
  Message Send2/1 -> Entity Output Switch2/1
  Simulink Function1/1(Out1) -> Message Send2/1
  Entity Server5/2 -> Entity Input Switch1/2
  Entity Output Switch2/1 -> Entity Input Switch1/1
  Constant1/1 -> Entity Server5/1
  Entity Server6/1 -> Entity Server5/2
  Entity Server7/1 -> VGR Moves from HBW to MPS/1
  Entity Server8/1 -> HBW ready to re-sort bin/1
  "   "/1 -> Entity Gate/2
